simulink model "Non_WindFarm"  (R2024a)
settings: Solver=ode45  StartTime=parSimulacio.ti  StopTime=200  MaxStep=parSimulacio.pas  RelTol=1e-6  AbsTol=1e-6  EnableMultiTasking=on
model workspace (MAT data in the model file):
  tt_vw : Simulink.Parameter (value not decoded)
values from neighbouring files (symbols this model uses):
  L = L'    [Lin_SignalGenerator.m]    (also in Non_ParameterInitialize.m; cal_QR.m = zeros(v, 1); parameters_windFarm2.m)
  nu = size(S, 1)    [Lin_SignalGenerator.m]    (also in Non_ParameterInitialize.m; parameters_windFarm2.m)
  S = zeros(v, v)    [cal_QR.m]
  w0 = [1 -0.00962521549583 0.0254779042049 -0.0160197396127 -0.0156056332727 0.0112137208272 0.0440607583301 -0.0193704893312 -0.0229464276306 -0.00247675309015 0.0285830611299]    [w0.mat]
undefined symbols (not defined in the file or in its folder): parControl, parConvertidor, parGenerador, parGrid, parMecanica, parSimulacio, windspeed
(part 39 of 40)

== system Non_WindFarm/FOM/Wind Farm/Wind Turbine Strings/String6/WT10/WFG/Maquina Sincrona/Park ==
  note: Page 24 eq 3.12
  theta_r : Inport
  Constant4 : Constant  Value=2*pi/3
  Gain7 : Gain  Gain=2/3
  Matrix Concatenate1 : Concatenate  NumInputs=3  Mode=Multidimensional array  ConcatenateDimension=2
  Matrix Concatenate2 : Concatenate  Mode=Multidimensional array  ConcatenateDimension=2
  Mux2 : Mux  Inputs=2
  Mux3 : Mux  Inputs=2
  Mux4 : Mux  Inputs=2
  Mux5 : Mux  Inputs=3
  Mux6 : Mux  Inputs=3
  Sum1 : Sum  Inputs=|++
  Sum2 : Sum  Inputs=|+-
  Trigonometric Function : Trigonometry  Operator=cos
  Trigonometric Function1 : Trigonometry
  Trigonometric Function2 : Trigonometry  Operator=cos
  Trigonometric Function3 : Trigonometry
  Trigonometric Function4 : Trigonometry  Operator=cos
  Trigonometric Function5 : Trigonometry
  Tthetar : Outport
  nTthetar : Outport  Port=2
  wires:
  Constant4/1 -> Sum2/2, Sum1/2
  Trigonometric Function/1 -> Mux2/1, Mux5/1
  Trigonometric Function1/1 -> Mux2/2, Mux6/1
  Trigonometric Function2/1 -> Mux3/1, Mux5/2
  Trigonometric Function3/1 -> Mux3/2, Mux6/2
  Trigonometric Function4/1 -> Mux4/1, Mux5/3
  Trigonometric Function5/1 -> Mux4/2, Mux6/3
  Mux2/1 -> Matrix Concatenate1/1
  Mux3/1 -> Matrix Concatenate1/2
  Mux4/1 -> Matrix Concatenate1/3
  Matrix Concatenate1/1 -> Gain7/1
  Mux5/1 -> Matrix Concatenate2/1
  Mux6/1 -> Matrix Concatenate2/2
  Gain7/1 -> Tthetar/1
  Matrix Concatenate2/1 -> nTthetar/1
  theta_r/1 -> Sum1/1, Sum2/1, Trigonometric Function1/1, Trigonometric Function/1
  Sum2/1 -> Trigonometric Function3/1, Trigonometric Function2/1
  Sum1/1 -> Trigonometric Function5/1, Trigonometric Function4/1

== system Non_WindFarm/FOM/Wind Farm/Wind Turbine Strings/String6/WT10/WFG/Mecanica nolineal i vent/Turbina ==
  note: Page 8
  note: Gamma_t-Wind turbine torque
  note: Wt-turbine speed
  note: Vw-wind speed
  note: Beta-pitch angle
  velocitat_vent : Inport
  omega_aleps : Inport  Port=2
  theta_aleps : Inport  Port=3
  Calcula_Cp : Fcn  Expr=c1*(c2*u[1]-c3*u[2]-c4*u[2]^c5-c6)*exp(-c7*u[1])
  Calcula_parell : Fcn  Expr=u[1]*rho*A*u[2]^3/(2*u[3])
  LAMBDA_inversa : Fcn  Expr=1/(u[1]+c8*u[2])-c9/(1+u[2]^3)
  Mux : Mux  Inputs=2
  Mux1 : Mux  Inputs=2
  Mux2 : Mux  Inputs=2
  Mux3 : Mux  Inputs=3
  calcula_lambda : Fcn  Expr=u[2]*R/u[1]
  parell_turbina : Outport
  Cp : Outport  Port=2
  wires:
  Mux1/1 -> calcula_lambda/1
  omega_aleps/1 -> Mux1/2, Mux3/3
  velocitat_vent/1 -> Mux1/1, Mux3/2
  calcula_lambda/1 -> Mux/1
  theta_aleps/1 -> Mux/2, Mux2/2
  Mux/1 -> LAMBDA_inversa/1
  LAMBDA_inversa/1 -> Mux2/1
  Mux2/1 -> Calcula_Cp/1
  Calcula_Cp/1 -> Mux3/1, Cp/1
  Mux3/1 -> Calcula_parell/1
  Calcula_parell/1 -> parell_turbina/1

== system Non_WindFarm/FOM/Wind Farm/Wind Turbine Strings/String6/WT2/Transformer-complex/homopolar sequence/Park ==
  theta_r : Inport
  Constant4 : Constant  Value=2*pi/3
  Gain7 : Gain  Gain=2/3
  Matrix Concatenate1 : Concatenate  NumInputs=3  Mode=Multidimensional array  ConcatenateDimension=2
  Matrix Concatenate2 : Concatenate  Mode=Multidimensional array  ConcatenateDimension=2
  Mux2 : Mux  Inputs=2
  Mux3 : Mux  Inputs=2
  Mux4 : Mux  Inputs=2
  Mux5 : Mux  Inputs=3
  Mux6 : Mux  Inputs=3
  Sum1 : Sum  Inputs=|++
  Sum2 : Sum  Inputs=|+-
  Trigonometric Function : Trigonometry  Operator=cos
  Trigonometric Function1 : Trigonometry
  Trigonometric Function2 : Trigonometry  Operator=cos
  Trigonometric Function3 : Trigonometry
  Trigonometric Function4 : Trigonometry  Operator=cos
  Trigonometric Function5 : Trigonometry
  Tthetar : Outport
  nTthetar : Outport  Port=2
  wires:
  theta_r/1 -> Sum1/1, Sum2/1, Trigonometric Function/1, Trigonometric Function1/1
  Sum2/1 -> Trigonometric Function2/1, Trigonometric Function3/1
  Sum1/1 -> Trigonometric Function4/1, Trigonometric Function5/1
  Constant4/1 -> Sum2/2, Sum1/2
  Trigonometric Function/1 -> Mux2/1, Mux5/1
  Trigonometric Function1/1 -> Mux2/2, Mux6/1
  Trigonometric Function2/1 -> Mux3/1, Mux5/2
  Trigonometric Function3/1 -> Mux3/2, Mux6/2
  Trigonometric Function4/1 -> Mux4/1, Mux5/3
  Trigonometric Function5/1 -> Mux4/2, Mux6/3
  Mux2/1 -> Matrix Concatenate1/1
  Mux3/1 -> Matrix Concatenate1/2
  Mux4/1 -> Matrix Concatenate1/3
  Matrix Concatenate1/1 -> Gain7/1
  Mux5/1 -> Matrix Concatenate2/1
  Mux6/1 -> Matrix Concatenate2/2
  Gain7/1 -> Tthetar/1
  Matrix Concatenate2/1 -> nTthetar/1

== system Non_WindFarm/FOM/Wind Farm/Wind Turbine Strings/String6/WT2/Transformer-complex/homopolar sequence/homopolar sequence 1 ==
  note: 1/3*v0
  v : Inport
  Add5 : Sum  Inputs=-+
  Constant : Constant  Value=1/3*ones(3)
  Product3 : Product  Multiplication=Matrix(*)  RndMeth=Zero
  v_bar : Outport
  wires:
  Add5/1 -> v_bar/1
  Product3/1 -> Add5/1
  Constant/1 -> Product3/1
  v/1 -> Product3/2, Add5/2

== system Non_WindFarm/FOM/Wind Farm/Wind Turbine Strings/String6/WT2/Transformer-complex/homopolar sequence/homopolar sequence 2 ==
  note: 1/3*v0
  v : Inport
  Add5 : Sum  Inputs=-+
  Constant : Constant  Value=[1/9,1/9,1/9;1/9,1/9,1/9;1/9,1/9,1/9]
  Product3 : Product  Multiplication=Matrix(*)  RndMeth=Zero
  v_bar : Outport
  wires:
  Add5/1 -> v_bar/1
  Product3/1 -> Add5/1
  Constant/1 -> Product3/1
  v/1 -> Product3/2, Add5/2

== system Non_WindFarm/FOM/Wind Farm/Wind Turbine Strings/String6/WT2/WFG/Control Electric Generador/PI ==
  e : Inport
  Demux : Demux  Outputs=2
  Mux2 : Mux  Inputs=2
  Transfer Fcn : TransferFcn  Numerator=[qKp qKi]  Denominator=[1 0]
  Transfer Fcn1 : TransferFcn  Numerator=[dKp dKi]  Denominator=[1 0]
  u : Outport
  wires:
  Transfer Fcn/1 -> Mux2/1
  Transfer Fcn1/1 -> Mux2/2
  Demux/1 -> Transfer Fcn/1
  Demux/2 -> Transfer Fcn1/1
  e/1 -> Demux/1
  Mux2/1 -> u/1

== system Non_WindFarm/FOM/Wind Farm/Wind Turbine Strings/String6/WT2/WFG/Control Electric Generador/Park ==
  theta_r : Inport
  Constant4 : Constant  Value=2*pi/3
  Gain7 : Gain  Gain=2/3
  Matrix Concatenate1 : Concatenate  NumInputs=3  Mode=Multidimensional array  ConcatenateDimension=2
  Matrix Concatenate2 : Concatenate  Mode=Multidimensional array  ConcatenateDimension=2
  Mux2 : Mux  Inputs=2
  Mux3 : Mux  Inputs=2
  Mux4 : Mux  Inputs=2
  Mux5 : Mux  Inputs=3
  Mux6 : Mux  Inputs=3
  Sum1 : Sum  Inputs=|++
  Sum2 : Sum  Inputs=|+-
  Trigonometric Function : Trigonometry  Operator=cos
  Trigonometric Function1 : Trigonometry
  Trigonometric Function2 : Trigonometry  Operator=cos
  Trigonometric Function3 : Trigonometry
  Trigonometric Function4 : Trigonometry  Operator=cos
  Trigonometric Function5 : Trigonometry
  Tthetar : Outport
  nTthetar : Outport  Port=2
  wires:
  theta_r/1 -> Sum1/1, Sum2/1, Trigonometric Function/1, Trigonometric Function1/1
  Sum2/1 -> Trigonometric Function2/1, Trigonometric Function3/1
  Sum1/1 -> Trigonometric Function4/1, Trigonometric Function5/1
  Constant4/1 -> Sum2/2, Sum1/2
  Trigonometric Function/1 -> Mux2/1, Mux5/1
  Trigonometric Function1/1 -> Mux2/2, Mux6/1
  Trigonometric Function2/1 -> Mux3/1, Mux5/2
  Trigonometric Function3/1 -> Mux3/2, Mux6/2
  Trigonometric Function4/1 -> Mux4/1, Mux5/3
  Trigonometric Function5/1 -> Mux4/2, Mux6/3
  Mux2/1 -> Matrix Concatenate1/1
  Mux3/1 -> Matrix Concatenate1/2
  Mux4/1 -> Matrix Concatenate1/3
  Matrix Concatenate1/1 -> Gain7/1
  Mux5/1 -> Matrix Concatenate2/1
  Mux6/1 -> Matrix Concatenate2/2
  Gain7/1 -> Tthetar/1
  Matrix Concatenate2/1 -> nTthetar/1

== system Non_WindFarm/FOM/Wind Farm/Wind Turbine Strings/String6/WT2/WFG/Control Electric Generador/Sat inf ==
  in : Inport
  Abs : Abs  SaturateOnIntegerOverflow=off
  Constant3 : Constant  Value=0.01
  Relational Operator : RelationalOperator  Operator=>  OutDataTypeStr=boolean  InputSameDT=off
  Switch : Switch  Criteria=u2 > Threshold  SaturateOnIntegerOverflow=off  InputSameDT=off
  out : Outport
  wires:
  Abs/1 -> Relational Operator/1
  Constant3/1 -> Relational Operator/2, Switch/3
  Relational Operator/1 -> Switch/2
  in/1 -> Abs/1, Switch/1
  Switch/1 -> out/1

== system Non_WindFarm/FOM/Wind Farm/Wind Turbine Strings/String6/WT2/WFG/Control de Corrent de Xarxa2/PI_d ==
  e : Inport
  Demux : Demux  Outputs=2
  Mux2 : Mux  Inputs=2
  Transfer Fcn : TransferFcn  Numerator=[Kp Ki]  Denominator=[1,0]
  Transfer Fcn1 : TransferFcn  Numerator=[Kp Ki]  Denominator=[1,0]
  u : Outport
  wires:
  Transfer Fcn/1 -> Mux2/1
  Transfer Fcn1/1 -> Mux2/2
  Demux/1 -> Transfer Fcn/1
  Demux/2 -> Transfer Fcn1/1
  e/1 -> Demux/1
  Mux2/1 -> u/1

== system Non_WindFarm/FOM/Wind Farm/Wind Turbine Strings/String6/WT2/WFG/Control de Corrent de Xarxa2/rotacio1 ==
  theta : Inport
  Constant1 : Constant  Value=2*pi/3
  Gain1 : Gain  Gain=-1
  Matrix Concatenate1 : Concatenate  Mode=Multidimensional array  ConcatenateDimension=2
  Matrix Concatenate2 : Concatenate  Mode=Multidimensional array  ConcatenateDimension=2
  Mux1 : Mux  Inputs=3
  Mux2 : Mux  Inputs=2
  Mux3 : Mux  Inputs=2
  Mux5 : Mux  Inputs=3
  Sum4 : Sum  Inputs=|+-
  Sum5 : Sum  Inputs=|++
  Sum6 : Sum  Inputs=|+-
  Sum7 : Sum  Inputs=|++
  Trigonometric Function{,6,8,10} (4 alike) : Trigonometry  Operator=cos
  Trigonometric Function{1,7,9,11} (4 alike) : Trigonometry
  T : Outport
  nT : Outport  Port=2
  wires:
  Trigonometric Function/1 -> Mux2/1, Mux3/2
  Trigonometric Function1/1 -> Gain1/1, Mux2/2
  Mux2/1 -> Matrix Concatenate1/1
  Mux3/1 -> Matrix Concatenate1/2
  Matrix Concatenate1/1 -> T/1
  Matrix Concatenate2/1 -> nT/1
  theta/1 -> Trigonometric Function6/1, Sum4/1, Sum5/1, Trigonometric Function9/1, Sum6/1, Sum7/1, Trigonometric Function/1, Trigonometric Function1/1
  Sum4/1 -> Trigonometric Function10/1
  Constant1/1 -> Sum4/2, Sum5/2, Sum6/2, Sum7/2
  Sum5/1 -> Trigonometric Function8/1
  Sum6/1 -> Trigonometric Function7/1
  Sum7/1 -> Trigonometric Function11/1
  Trigonometric Function6/1 -> Mux5/1
  Trigonometric Function10/1 -> Mux5/2
  Trigonometric Function8/1 -> Mux5/3
  Trigonometric Function9/1 -> Mux1/1
  Trigonometric Function7/1 -> Mux1/2
  Trigonometric Function11/1 -> Mux1/3
  Mux5/1 -> Matrix Concatenate2/1
  Mux1/1 -> Matrix Concatenate2/2
  Gain1/1 -> Mux3/1

== system Non_WindFarm/FOM/Wind Farm/Wind Turbine Strings/String6/WT2/WFG/Maquina Sincrona/Park ==
  note: Page 24 eq 3.12
  theta_r : Inport
  Constant4 : Constant  Value=2*pi/3
  Gain7 : Gain  Gain=2/3
  Matrix Concatenate1 : Concatenate  NumInputs=3  Mode=Multidimensional array  ConcatenateDimension=2
  Matrix Concatenate2 : Concatenate  Mode=Multidimensional array  ConcatenateDimension=2
  Mux2 : Mux  Inputs=2
  Mux3 : Mux  Inputs=2
  Mux4 : Mux  Inputs=2
  Mux5 : Mux  Inputs=3
  Mux6 : Mux  Inputs=3
  Sum1 : Sum  Inputs=|++
  Sum2 : Sum  Inputs=|+-
  Trigonometric Function : Trigonometry  Operator=cos
  Trigonometric Function1 : Trigonometry
  Trigonometric Function2 : Trigonometry  Operator=cos
  Trigonometric Function3 : Trigonometry
  Trigonometric Function4 : Trigonometry  Operator=cos
  Trigonometric Function5 : Trigonometry
  Tthetar : Outport
  nTthetar : Outport  Port=2
  wires:
  Constant4/1 -> Sum2/2, Sum1/2
  Trigonometric Function/1 -> Mux2/1, Mux5/1
  Trigonometric Function1/1 -> Mux2/2, Mux6/1
  Trigonometric Function2/1 -> Mux3/1, Mux5/2
  Trigonometric Function3/1 -> Mux3/2, Mux6/2
  Trigonometric Function4/1 -> Mux4/1, Mux5/3
  Trigonometric Function5/1 -> Mux4/2, Mux6/3
  Mux2/1 -> Matrix Concatenate1/1
  Mux3/1 -> Matrix Concatenate1/2
  Mux4/1 -> Matrix Concatenate1/3
  Matrix Concatenate1/1 -> Gain7/1
  Mux5/1 -> Matrix Concatenate2/1
  Mux6/1 -> Matrix Concatenate2/2
  Gain7/1 -> Tthetar/1
  Matrix Concatenate2/1 -> nTthetar/1
  theta_r/1 -> Sum1/1, Sum2/1, Trigonometric Function1/1, Trigonometric Function/1
  Sum2/1 -> Trigonometric Function3/1, Trigonometric Function2/1
  Sum1/1 -> Trigonometric Function5/1, Trigonometric Function4/1

== system Non_WindFarm/FOM/Wind Farm/Wind Turbine Strings/String6/WT2/WFG/Mecanica nolineal i vent/Turbina ==
  note: Page 8
  note: Gamma_t-Wind turbine torque
  note: Wt-turbine speed
  note: Vw-wind speed
  note: Beta-pitch angle
  velocitat_vent : Inport
  omega_aleps : Inport  Port=2
  theta_aleps : Inport  Port=3
  Calcula_Cp : Fcn  Expr=c1*(c2*u[1]-c3*u[2]-c4*u[2]^c5-c6)*exp(-c7*u[1])
  Calcula_parell : Fcn  Expr=u[1]*rho*A*u[2]^3/(2*u[3])
  LAMBDA_inversa : Fcn  Expr=1/(u[1]+c8*u[2])-c9/(1+u[2]^3)
  Mux : Mux  Inputs=2
  Mux1 : Mux  Inputs=2
  Mux2 : Mux  Inputs=2
  Mux3 : Mux  Inputs=3
  calcula_lambda : Fcn  Expr=u[2]*R/u[1]
  parell_turbina : Outport
  Cp : Outport  Port=2
  wires:
  Mux1/1 -> calcula_lambda/1
  omega_aleps/1 -> Mux1/2, Mux3/3
  velocitat_vent/1 -> Mux1/1, Mux3/2
  calcula_lambda/1 -> Mux/1
  theta_aleps/1 -> Mux/2, Mux2/2
  Mux/1 -> LAMBDA_inversa/1
  LAMBDA_inversa/1 -> Mux2/1
  Mux2/1 -> Calcula_Cp/1
  Calcula_Cp/1 -> Mux3/1, Cp/1
  Mux3/1 -> Calcula_parell/1
  Calcula_parell/1 -> parell_turbina/1

== system Non_WindFarm/FOM/Wind Farm/Wind Turbine Strings/String6/WT3/Transformer-complex/homopolar sequence/Park ==
  theta_r : Inport
  Constant4 : Constant  Value=2*pi/3
  Gain7 : Gain  Gain=2/3
  Matrix Concatenate1 : Concatenate  NumInputs=3  Mode=Multidimensional array  ConcatenateDimension=2
  Matrix Concatenate2 : Concatenate  Mode=Multidimensional array  ConcatenateDimension=2
  Mux2 : Mux  Inputs=2
  Mux3 : Mux  Inputs=2
  Mux4 : Mux  Inputs=2
  Mux5 : Mux  Inputs=3
  Mux6 : Mux  Inputs=3
  Sum1 : Sum  Inputs=|++
  Sum2 : Sum  Inputs=|+-
  Trigonometric Function : Trigonometry  Operator=cos
  Trigonometric Function1 : Trigonometry
  Trigonometric Function2 : Trigonometry  Operator=cos
  Trigonometric Function3 : Trigonometry
  Trigonometric Function4 : Trigonometry  Operator=cos
  Trigonometric Function5 : Trigonometry
  Tthetar : Outport
  nTthetar : Outport  Port=2
  wires:
  Matrix Concatenate2/1 -> nTthetar/1
  Gain7/1 -> Tthetar/1
  Mux6/1 -> Matrix Concatenate2/2
  Mux5/1 -> Matrix Concatenate2/1
  Matrix Concatenate1/1 -> Gain7/1
  Mux4/1 -> Matrix Concatenate1/3
  Mux3/1 -> Matrix Concatenate1/2
  Mux2/1 -> Matrix Concatenate1/1
  Trigonometric Function5/1 -> Mux6/3, Mux4/2
  Trigonometric Function4/1 -> Mux5/3, Mux4/1
  Trigonometric Function3/1 -> Mux6/2, Mux3/2
  Trigonometric Function2/1 -> Mux5/2, Mux3/1
  Trigonometric Function1/1 -> Mux6/1, Mux2/2
  Trigonometric Function/1 -> Mux5/1, Mux2/1
  Constant4/1 -> Sum1/2, Sum2/2
  Sum1/1 -> Trigonometric Function5/1, Trigonometric Function4/1
  Sum2/1 -> Trigonometric Function3/1, Trigonometric Function2/1
  theta_r/1 -> Trigonometric Function1/1, Trigonometric Function/1, Sum2/1, Sum1/1

== system Non_WindFarm/FOM/Wind Farm/Wind Turbine Strings/String6/WT3/Transformer-complex/homopolar sequence/homopolar sequence 1 ==
  note: 1/3*v0
  v : Inport
  Add5 : Sum  Inputs=-+
  Constant : Constant  Value=1/3*ones(3)
  Product3 : Product  Multiplication=Matrix(*)  RndMeth=Zero
  v_bar : Outport
  wires:
  v/1 -> Add5/2, Product3/2
  Constant/1 -> Product3/1
  Product3/1 -> Add5/1
  Add5/1 -> v_bar/1

== system Non_WindFarm/FOM/Wind Farm/Wind Turbine Strings/String6/WT3/Transformer-complex/homopolar sequence/homopolar sequence 2 ==
  note: 1/3*v0
  v : Inport
  Add5 : Sum  Inputs=-+
  Constant : Constant  Value=[1/9,1/9,1/9;1/9,1/9,1/9;1/9,1/9,1/9]
  Product3 : Product  Multiplication=Matrix(*)  RndMeth=Zero
  v_bar : Outport
  wires:
  v/1 -> Add5/2, Product3/2
  Constant/1 -> Product3/1
  Product3/1 -> Add5/1
  Add5/1 -> v_bar/1

== system Non_WindFarm/FOM/Wind Farm/Wind Turbine Strings/String6/WT3/WFG/Control Electric Generador/PI ==
  e : Inport
  Demux : Demux  Outputs=2
  Mux2 : Mux  Inputs=2
  Transfer Fcn : TransferFcn  Numerator=[qKp qKi]  Denominator=[1 0]
  Transfer Fcn1 : TransferFcn  Numerator=[dKp dKi]  Denominator=[1 0]
  u : Outport
  wires:
  Transfer Fcn/1 -> Mux2/1
  Transfer Fcn1/1 -> Mux2/2
  Demux/1 -> Transfer Fcn/1
  Demux/2 -> Transfer Fcn1/1
  e/1 -> Demux/1
  Mux2/1 -> u/1

== system Non_WindFarm/FOM/Wind Farm/Wind Turbine Strings/String6/WT3/WFG/Control Electric Generador/Park ==
  theta_r : Inport
  Constant4 : Constant  Value=2*pi/3
  Gain7 : Gain  Gain=2/3
  Matrix Concatenate1 : Concatenate  NumInputs=3  Mode=Multidimensional array  ConcatenateDimension=2
  Matrix Concatenate2 : Concatenate  Mode=Multidimensional array  ConcatenateDimension=2
  Mux2 : Mux  Inputs=2
  Mux3 : Mux  Inputs=2
  Mux4 : Mux  Inputs=2
  Mux5 : Mux  Inputs=3
  Mux6 : Mux  Inputs=3
  Sum1 : Sum  Inputs=|++
  Sum2 : Sum  Inputs=|+-
  Trigonometric Function : Trigonometry  Operator=cos
  Trigonometric Function1 : Trigonometry
  Trigonometric Function2 : Trigonometry  Operator=cos
  Trigonometric Function3 : Trigonometry
  Trigonometric Function4 : Trigonometry  Operator=cos
  Trigonometric Function5 : Trigonometry
  Tthetar : Outport
  nTthetar : Outport  Port=2
  wires:
  theta_r/1 -> Sum1/1, Sum2/1, Trigonometric Function/1, Trigonometric Function1/1
  Sum2/1 -> Trigonometric Function2/1, Trigonometric Function3/1
  Sum1/1 -> Trigonometric Function4/1, Trigonometric Function5/1
  Constant4/1 -> Sum2/2, Sum1/2
  Trigonometric Function/1 -> Mux2/1, Mux5/1
  Trigonometric Function1/1 -> Mux2/2, Mux6/1
  Trigonometric Function2/1 -> Mux3/1, Mux5/2
  Trigonometric Function3/1 -> Mux3/2, Mux6/2
  Trigonometric Function4/1 -> Mux4/1, Mux5/3
  Trigonometric Function5/1 -> Mux4/2, Mux6/3
  Mux2/1 -> Matrix Concatenate1/1
  Mux3/1 -> Matrix Concatenate1/2
  Mux4/1 -> Matrix Concatenate1/3
  Matrix Concatenate1/1 -> Gain7/1
  Mux5/1 -> Matrix Concatenate2/1
  Mux6/1 -> Matrix Concatenate2/2
  Gain7/1 -> Tthetar/1
  Matrix Concatenate2/1 -> nTthetar/1

== system Non_WindFarm/FOM/Wind Farm/Wind Turbine Strings/String6/WT3/WFG/Control Electric Generador/Sat inf ==
  in : Inport
  Abs : Abs  SaturateOnIntegerOverflow=off
  Constant3 : Constant  Value=0.01
  Relational Operator : RelationalOperator  Operator=>  OutDataTypeStr=boolean  InputSameDT=off
  Switch : Switch  Criteria=u2 > Threshold  SaturateOnIntegerOverflow=off  InputSameDT=off
  out : Outport
  wires:
  Abs/1 -> Relational Operator/1
  Constant3/1 -> Relational Operator/2, Switch/3
  Relational Operator/1 -> Switch/2
  in/1 -> Abs/1, Switch/1
  Switch/1 -> out/1

== system Non_WindFarm/FOM/Wind Farm/Wind Turbine Strings/String6/WT3/WFG/Control de Corrent de Xarxa2/PI_d ==
  e : Inport
  Demux : Demux  Outputs=2
  Mux2 : Mux  Inputs=2
  Transfer Fcn : TransferFcn  Numerator=[Kp Ki]  Denominator=[1,0]
  Transfer Fcn1 : TransferFcn  Numerator=[Kp Ki]  Denominator=[1,0]
  u : Outport
  wires:
  Transfer Fcn/1 -> Mux2/1
  Transfer Fcn1/1 -> Mux2/2
  Demux/1 -> Transfer Fcn/1
  Demux/2 -> Transfer Fcn1/1
  e/1 -> Demux/1
  Mux2/1 -> u/1

== system Non_WindFarm/FOM/Wind Farm/Wind Turbine Strings/String6/WT3/WFG/Control de Corrent de Xarxa2/rotacio1 ==
  theta : Inport
  Constant1 : Constant  Value=2*pi/3
  Gain1 : Gain  Gain=-1
  Matrix Concatenate1 : Concatenate  Mode=Multidimensional array  ConcatenateDimension=2
  Matrix Concatenate2 : Concatenate  Mode=Multidimensional array  ConcatenateDimension=2
  Mux1 : Mux  Inputs=3
  Mux2 : Mux  Inputs=2
  Mux3 : Mux  Inputs=2
  Mux5 : Mux  Inputs=3
  Sum4 : Sum  Inputs=|+-
  Sum5 : Sum  Inputs=|++
  Sum6 : Sum  Inputs=|+-
  Sum7 : Sum  Inputs=|++
  Trigonometric Function{,6,8,10} (4 alike) : Trigonometry  Operator=cos
  Trigonometric Function{1,7,9,11} (4 alike) : Trigonometry
  T : Outport
  nT : Outport  Port=2
  wires:
  Trigonometric Function/1 -> Mux2/1, Mux3/2
  Trigonometric Function1/1 -> Gain1/1, Mux2/2
  Mux2/1 -> Matrix Concatenate1/1
  Mux3/1 -> Matrix Concatenate1/2
  Matrix Concatenate1/1 -> T/1
  Matrix Concatenate2/1 -> nT/1
  theta/1 -> Trigonometric Function6/1, Sum4/1, Sum5/1, Trigonometric Function9/1, Sum6/1, Sum7/1, Trigonometric Function/1, Trigonometric Function1/1
  Sum4/1 -> Trigonometric Function10/1
  Constant1/1 -> Sum4/2, Sum5/2, Sum6/2, Sum7/2
  Sum5/1 -> Trigonometric Function8/1
  Sum6/1 -> Trigonometric Function7/1
  Sum7/1 -> Trigonometric Function11/1
  Trigonometric Function6/1 -> Mux5/1
  Trigonometric Function10/1 -> Mux5/2
  Trigonometric Function8/1 -> Mux5/3
  Trigonometric Function9/1 -> Mux1/1
  Trigonometric Function7/1 -> Mux1/2
  Trigonometric Function11/1 -> Mux1/3
  Mux5/1 -> Matrix Concatenate2/1
  Mux1/1 -> Matrix Concatenate2/2
  Gain1/1 -> Mux3/1

== system Non_WindFarm/FOM/Wind Farm/Wind Turbine Strings/String6/WT3/WFG/Maquina Sincrona/Park ==
  note: Page 24 eq 3.12
  theta_r : Inport
  Constant4 : Constant  Value=2*pi/3
  Gain7 : Gain  Gain=2/3
  Matrix Concatenate1 : Concatenate  NumInputs=3  Mode=Multidimensional array  ConcatenateDimension=2
  Matrix Concatenate2 : Concatenate  Mode=Multidimensional array  ConcatenateDimension=2
  Mux2 : Mux  Inputs=2
  Mux3 : Mux  Inputs=2
  Mux4 : Mux  Inputs=2
  Mux5 : Mux  Inputs=3
  Mux6 : Mux  Inputs=3
  Sum1 : Sum  Inputs=|++
  Sum2 : Sum  Inputs=|+-
  Trigonometric Function : Trigonometry  Operator=cos
  Trigonometric Function1 : Trigonometry
  Trigonometric Function2 : Trigonometry  Operator=cos
  Trigonometric Function3 : Trigonometry
  Trigonometric Function4 : Trigonometry  Operator=cos
  Trigonometric Function5 : Trigonometry
  Tthetar : Outport
  nTthetar : Outport  Port=2
  wires:
  Constant4/1 -> Sum2/2, Sum1/2
  Trigonometric Function/1 -> Mux2/1, Mux5/1
  Trigonometric Function1/1 -> Mux2/2, Mux6/1
  Trigonometric Function2/1 -> Mux3/1, Mux5/2
  Trigonometric Function3/1 -> Mux3/2, Mux6/2
  Trigonometric Function4/1 -> Mux4/1, Mux5/3
  Trigonometric Function5/1 -> Mux4/2, Mux6/3
  Mux2/1 -> Matrix Concatenate1/1
  Mux3/1 -> Matrix Concatenate1/2
  Mux4/1 -> Matrix Concatenate1/3
  Matrix Concatenate1/1 -> Gain7/1
  Mux5/1 -> Matrix Concatenate2/1
  Mux6/1 -> Matrix Concatenate2/2
  Gain7/1 -> Tthetar/1
  Matrix Concatenate2/1 -> nTthetar/1
  theta_r/1 -> Sum1/1, Sum2/1, Trigonometric Function1/1, Trigonometric Function/1
  Sum2/1 -> Trigonometric Function3/1, Trigonometric Function2/1
  Sum1/1 -> Trigonometric Function5/1, Trigonometric Function4/1

== system Non_WindFarm/FOM/Wind Farm/Wind Turbine Strings/String6/WT3/WFG/Mecanica nolineal i vent/Turbina ==
  note: Page 8
  note: Gamma_t-Wind turbine torque
  note: Wt-turbine speed
  note: Vw-wind speed
  note: Beta-pitch angle
  velocitat_vent : Inport
  omega_aleps : Inport  Port=2
  theta_aleps : Inport  Port=3
  Calcula_Cp : Fcn  Expr=c1*(c2*u[1]-c3*u[2]-c4*u[2]^c5-c6)*exp(-c7*u[1])
  Calcula_parell : Fcn  Expr=u[1]*rho*A*u[2]^3/(2*u[3])
  LAMBDA_inversa : Fcn  Expr=1/(u[1]+c8*u[2])-c9/(1+u[2]^3)
  Mux : Mux  Inputs=2
  Mux1 : Mux  Inputs=2
  Mux2 : Mux  Inputs=2
  Mux3 : Mux  Inputs=3
  calcula_lambda : Fcn  Expr=u[2]*R/u[1]
  parell_turbina : Outport
  Cp : Outport  Port=2
  wires:
  Mux1/1 -> calcula_lambda/1
  omega_aleps/1 -> Mux1/2, Mux3/3
  velocitat_vent/1 -> Mux1/1, Mux3/2
  calcula_lambda/1 -> Mux/1
  theta_aleps/1 -> Mux/2, Mux2/2
  Mux/1 -> LAMBDA_inversa/1
  LAMBDA_inversa/1 -> Mux2/1
  Mux2/1 -> Calcula_Cp/1
  Calcula_Cp/1 -> Mux3/1, Cp/1
  Mux3/1 -> Calcula_parell/1
  Calcula_parell/1 -> parell_turbina/1

== system Non_WindFarm/FOM/Wind Farm/Wind Turbine Strings/String6/WT4/Transformer-complex/homopolar sequence/Park ==
  theta_r : Inport
  Constant4 : Constant  Value=2*pi/3
  Gain7 : Gain  Gain=2/3
  Matrix Concatenate1 : Concatenate  NumInputs=3  Mode=Multidimensional array  ConcatenateDimension=2
  Matrix Concatenate2 : Concatenate  Mode=Multidimensional array  ConcatenateDimension=2
  Mux2 : Mux  Inputs=2
  Mux3 : Mux  Inputs=2
  Mux4 : Mux  Inputs=2
  Mux5 : Mux  Inputs=3
  Mux6 : Mux  Inputs=3
  Sum1 : Sum  Inputs=|++
  Sum2 : Sum  Inputs=|+-
  Trigonometric Function : Trigonometry  Operator=cos
  Trigonometric Function1 : Trigonometry
  Trigonometric Function2 : Trigonometry  Operator=cos
  Trigonometric Function3 : Trigonometry
  Trigonometric Function4 : Trigonometry  Operator=cos
  Trigonometric Function5 : Trigonometry
  Tthetar : Outport
  nTthetar : Outport  Port=2
  wires:
  theta_r/1 -> Sum1/1, Sum2/1, Trigonometric Function/1, Trigonometric Function1/1
  Sum2/1 -> Trigonometric Function2/1, Trigonometric Function3/1
  Sum1/1 -> Trigonometric Function4/1, Trigonometric Function5/1
  Constant4/1 -> Sum2/2, Sum1/2
  Trigonometric Function/1 -> Mux2/1, Mux5/1
  Trigonometric Function1/1 -> Mux2/2, Mux6/1
  Trigonometric Function2/1 -> Mux3/1, Mux5/2
  Trigonometric Function3/1 -> Mux3/2, Mux6/2
  Trigonometric Function4/1 -> Mux4/1, Mux5/3
  Trigonometric Function5/1 -> Mux4/2, Mux6/3
  Mux2/1 -> Matrix Concatenate1/1
  Mux3/1 -> Matrix Concatenate1/2
  Mux4/1 -> Matrix Concatenate1/3
  Matrix Concatenate1/1 -> Gain7/1
  Mux5/1 -> Matrix Concatenate2/1
  Mux6/1 -> Matrix Concatenate2/2
  Gain7/1 -> Tthetar/1
  Matrix Concatenate2/1 -> nTthetar/1

== system Non_WindFarm/FOM/Wind Farm/Wind Turbine Strings/String6/WT4/Transformer-complex/homopolar sequence/homopolar sequence 1 ==
  note: 1/3*v0
  v : Inport
  Add5 : Sum  Inputs=-+
  Constant : Constant  Value=1/3*ones(3)
  Product3 : Product  Multiplication=Matrix(*)  RndMeth=Zero
  v_bar : Outport
  wires:
  Add5/1 -> v_bar/1
  Product3/1 -> Add5/1
  Constant/1 -> Product3/1
  v/1 -> Product3/2, Add5/2

== system Non_WindFarm/FOM/Wind Farm/Wind Turbine Strings/String6/WT4/Transformer-complex/homopolar sequence/homopolar sequence 2 ==
  note: 1/3*v0
  v : Inport
  Add5 : Sum  Inputs=-+
  Constant : Constant  Value=[1/9,1/9,1/9;1/9,1/9,1/9;1/9,1/9,1/9]
  Product3 : Product  Multiplication=Matrix(*)  RndMeth=Zero
  v_bar : Outport
  wires:
  Add5/1 -> v_bar/1
  Product3/1 -> Add5/1
  Constant/1 -> Product3/1
  v/1 -> Product3/2, Add5/2

== system Non_WindFarm/FOM/Wind Farm/Wind Turbine Strings/String6/WT4/WFG/Control Electric Generador/PI ==
  e : Inport
  Demux : Demux  Outputs=2
  Mux2 : Mux  Inputs=2
  Transfer Fcn : TransferFcn  Numerator=[qKp qKi]  Denominator=[1 0]
  Transfer Fcn1 : TransferFcn  Numerator=[dKp dKi]  Denominator=[1 0]
  u : Outport
  wires:
  Transfer Fcn/1 -> Mux2/1
  Transfer Fcn1/1 -> Mux2/2
  Demux/1 -> Transfer Fcn/1
  Demux/2 -> Transfer Fcn1/1
  e/1 -> Demux/1
  Mux2/1 -> u/1

== system Non_WindFarm/FOM/Wind Farm/Wind Turbine Strings/String6/WT4/WFG/Control Electric Generador/Park ==
  theta_r : Inport
  Constant4 : Constant  Value=2*pi/3
  Gain7 : Gain  Gain=2/3
  Matrix Concatenate1 : Concatenate  NumInputs=3  Mode=Multidimensional array  ConcatenateDimension=2
  Matrix Concatenate2 : Concatenate  Mode=Multidimensional array  ConcatenateDimension=2
  Mux2 : Mux  Inputs=2
  Mux3 : Mux  Inputs=2
  Mux4 : Mux  Inputs=2
  Mux5 : Mux  Inputs=3
  Mux6 : Mux  Inputs=3
  Sum1 : Sum  Inputs=|++
  Sum2 : Sum  Inputs=|+-
  Trigonometric Function : Trigonometry  Operator=cos
  Trigonometric Function1 : Trigonometry
  Trigonometric Function2 : Trigonometry  Operator=cos
  Trigonometric Function3 : Trigonometry
  Trigonometric Function4 : Trigonometry  Operator=cos
  Trigonometric Function5 : Trigonometry
  Tthetar : Outport
  nTthetar : Outport  Port=2
  wires:
  theta_r/1 -> Sum1/1, Sum2/1, Trigonometric Function/1, Trigonometric Function1/1
  Sum2/1 -> Trigonometric Function2/1, Trigonometric Function3/1
  Sum1/1 -> Trigonometric Function4/1, Trigonometric Function5/1
  Constant4/1 -> Sum2/2, Sum1/2
  Trigonometric Function/1 -> Mux2/1, Mux5/1
  Trigonometric Function1/1 -> Mux2/2, Mux6/1
  Trigonometric Function2/1 -> Mux3/1, Mux5/2
  Trigonometric Function3/1 -> Mux3/2, Mux6/2
  Trigonometric Function4/1 -> Mux4/1, Mux5/3
  Trigonometric Function5/1 -> Mux4/2, Mux6/3
  Mux2/1 -> Matrix Concatenate1/1
  Mux3/1 -> Matrix Concatenate1/2
  Mux4/1 -> Matrix Concatenate1/3
  Matrix Concatenate1/1 -> Gain7/1
  Mux5/1 -> Matrix Concatenate2/1
  Mux6/1 -> Matrix Concatenate2/2
  Gain7/1 -> Tthetar/1
  Matrix Concatenate2/1 -> nTthetar/1

== system Non_WindFarm/FOM/Wind Farm/Wind Turbine Strings/String6/WT4/WFG/Control Electric Generador/Sat inf ==
  in : Inport
  Abs : Abs  SaturateOnIntegerOverflow=off
  Constant3 : Constant  Value=0.01
  Relational Operator : RelationalOperator  Operator=>  OutDataTypeStr=boolean  InputSameDT=off
  Switch : Switch  Criteria=u2 > Threshold  SaturateOnIntegerOverflow=off  InputSameDT=off
  out : Outport
  wires:
  Abs/1 -> Relational Operator/1
  Constant3/1 -> Relational Operator/2, Switch/3
  Relational Operator/1 -> Switch/2
  in/1 -> Abs/1, Switch/1
  Switch/1 -> out/1

== system Non_WindFarm/FOM/Wind Farm/Wind Turbine Strings/String6/WT4/WFG/Control de Corrent de Xarxa2/PI_d ==
  e : Inport
  Demux : Demux  Outputs=2
  Mux2 : Mux  Inputs=2
  Transfer Fcn : TransferFcn  Numerator=[Kp Ki]  Denominator=[1,0]
  Transfer Fcn1 : TransferFcn  Numerator=[Kp Ki]  Denominator=[1,0]
  u : Outport
  wires:
  Transfer Fcn/1 -> Mux2/1
  Transfer Fcn1/1 -> Mux2/2
  Demux/1 -> Transfer Fcn/1
  Demux/2 -> Transfer Fcn1/1
  e/1 -> Demux/1
  Mux2/1 -> u/1

== system Non_WindFarm/FOM/Wind Farm/Wind Turbine Strings/String6/WT4/WFG/Control de Corrent de Xarxa2/rotacio1 ==
  theta : Inport
  Constant1 : Constant  Value=2*pi/3
  Gain1 : Gain  Gain=-1
  Matrix Concatenate1 : Concatenate  Mode=Multidimensional array  ConcatenateDimension=2
  Matrix Concatenate2 : Concatenate  Mode=Multidimensional array  ConcatenateDimension=2
  Mux1 : Mux  Inputs=3
  Mux2 : Mux  Inputs=2
  Mux3 : Mux  Inputs=2
  Mux5 : Mux  Inputs=3
  Sum4 : Sum  Inputs=|+-
  Sum5 : Sum  Inputs=|++
  Sum6 : Sum  Inputs=|+-
  Sum7 : Sum  Inputs=|++
  Trigonometric Function{,6,8,10} (4 alike) : Trigonometry  Operator=cos
  Trigonometric Function{1,7,9,11} (4 alike) : Trigonometry
  T : Outport
  nT : Outport  Port=2
  wires:
  Trigonometric Function/1 -> Mux2/1, Mux3/2
  Trigonometric Function1/1 -> Gain1/1, Mux2/2
  Mux2/1 -> Matrix Concatenate1/1
  Mux3/1 -> Matrix Concatenate1/2
  Matrix Concatenate1/1 -> T/1
  Matrix Concatenate2/1 -> nT/1
  theta/1 -> Trigonometric Function6/1, Sum4/1, Sum5/1, Trigonometric Function9/1, Sum6/1, Sum7/1, Trigonometric Function/1, Trigonometric Function1/1
  Sum4/1 -> Trigonometric Function10/1
  Constant1/1 -> Sum4/2, Sum5/2, Sum6/2, Sum7/2
  Sum5/1 -> Trigonometric Function8/1
  Sum6/1 -> Trigonometric Function7/1
  Sum7/1 -> Trigonometric Function11/1
  Trigonometric Function6/1 -> Mux5/1
  Trigonometric Function10/1 -> Mux5/2
  Trigonometric Function8/1 -> Mux5/3
  Trigonometric Function9/1 -> Mux1/1
  Trigonometric Function7/1 -> Mux1/2
  Trigonometric Function11/1 -> Mux1/3
  Mux5/1 -> Matrix Concatenate2/1
  Mux1/1 -> Matrix Concatenate2/2
  Gain1/1 -> Mux3/1

== system Non_WindFarm/FOM/Wind Farm/Wind Turbine Strings/String6/WT4/WFG/Maquina Sincrona/Park ==
  note: Page 24 eq 3.12
  theta_r : Inport
  Constant4 : Constant  Value=2*pi/3
  Gain7 : Gain  Gain=2/3
  Matrix Concatenate1 : Concatenate  NumInputs=3  Mode=Multidimensional array  ConcatenateDimension=2
  Matrix Concatenate2 : Concatenate  Mode=Multidimensional array  ConcatenateDimension=2
  Mux2 : Mux  Inputs=2
  Mux3 : Mux  Inputs=2
  Mux4 : Mux  Inputs=2
  Mux5 : Mux  Inputs=3
  Mux6 : Mux  Inputs=3
  Sum1 : Sum  Inputs=|++
  Sum2 : Sum  Inputs=|+-
  Trigonometric Function : Trigonometry  Operator=cos
  Trigonometric Function1 : Trigonometry
  Trigonometric Function2 : Trigonometry  Operator=cos
  Trigonometric Function3 : Trigonometry
  Trigonometric Function4 : Trigonometry  Operator=cos
  Trigonometric Function5 : Trigonometry
  Tthetar : Outport
  nTthetar : Outport  Port=2
  wires:
  Constant4/1 -> Sum2/2, Sum1/2
  Trigonometric Function/1 -> Mux2/1, Mux5/1
  Trigonometric Function1/1 -> Mux2/2, Mux6/1
  Trigonometric Function2/1 -> Mux3/1, Mux5/2
  Trigonometric Function3/1 -> Mux3/2, Mux6/2
  Trigonometric Function4/1 -> Mux4/1, Mux5/3
  Trigonometric Function5/1 -> Mux4/2, Mux6/3
  Mux2/1 -> Matrix Concatenate1/1
  Mux3/1 -> Matrix Concatenate1/2
  Mux4/1 -> Matrix Concatenate1/3
  Matrix Concatenate1/1 -> Gain7/1
  Mux5/1 -> Matrix Concatenate2/1
  Mux6/1 -> Matrix Concatenate2/2
  Gain7/1 -> Tthetar/1
  Matrix Concatenate2/1 -> nTthetar/1
  theta_r/1 -> Sum1/1, Sum2/1, Trigonometric Function1/1, Trigonometric Function/1
  Sum2/1 -> Trigonometric Function3/1, Trigonometric Function2/1
  Sum1/1 -> Trigonometric Function5/1, Trigonometric Function4/1

== system Non_WindFarm/FOM/Wind Farm/Wind Turbine Strings/String6/WT4/WFG/Mecanica nolineal i vent/Turbina ==
  note: Page 8
  note: Gamma_t-Wind turbine torque
  note: Wt-turbine speed
  note: Vw-wind speed
  note: Beta-pitch angle
  velocitat_vent : Inport
  omega_aleps : Inport  Port=2
  theta_aleps : Inport  Port=3
  Calcula_Cp : Fcn  Expr=c1*(c2*u[1]-c3*u[2]-c4*u[2]^c5-c6)*exp(-c7*u[1])
  Calcula_parell : Fcn  Expr=u[1]*rho*A*u[2]^3/(2*u[3])
  LAMBDA_inversa : Fcn  Expr=1/(u[1]+c8*u[2])-c9/(1+u[2]^3)
  Mux : Mux  Inputs=2
  Mux1 : Mux  Inputs=2
  Mux2 : Mux  Inputs=2
  Mux3 : Mux  Inputs=3
  calcula_lambda : Fcn  Expr=u[2]*R/u[1]
  parell_turbina : Outport
  Cp : Outport  Port=2
  wires:
  Mux1/1 -> calcula_lambda/1
  omega_aleps/1 -> Mux1/2, Mux3/3
  velocitat_vent/1 -> Mux1/1, Mux3/2
  calcula_lambda/1 -> Mux/1
  theta_aleps/1 -> Mux/2, Mux2/2
  Mux/1 -> LAMBDA_inversa/1
  LAMBDA_inversa/1 -> Mux2/1
  Mux2/1 -> Calcula_Cp/1
  Calcula_Cp/1 -> Mux3/1, Cp/1
  Mux3/1 -> Calcula_parell/1
  Calcula_parell/1 -> parell_turbina/1

== system Non_WindFarm/FOM/Wind Farm/Wind Turbine Strings/String6/WT5/Transformer-complex/homopolar sequence/Park ==
  theta_r : Inport
  Constant4 : Constant  Value=2*pi/3
  Gain7 : Gain  Gain=2/3
  Matrix Concatenate1 : Concatenate  NumInputs=3  Mode=Multidimensional array  ConcatenateDimension=2
  Matrix Concatenate2 : Concatenate  Mode=Multidimensional array  ConcatenateDimension=2
  Mux2 : Mux  Inputs=2
  Mux3 : Mux  Inputs=2
  Mux4 : Mux  Inputs=2
  Mux5 : Mux  Inputs=3
  Mux6 : Mux  Inputs=3
  Sum1 : Sum  Inputs=|++
  Sum2 : Sum  Inputs=|+-
  Trigonometric Function : Trigonometry  Operator=cos
  Trigonometric Function1 : Trigonometry
  Trigonometric Function2 : Trigonometry  Operator=cos
  Trigonometric Function3 : Trigonometry
  Trigonometric Function4 : Trigonometry  Operator=cos
  Trigonometric Function5 : Trigonometry
  Tthetar : Outport
  nTthetar : Outport  Port=2
  wires:
  Matrix Concatenate2/1 -> nTthetar/1
  Gain7/1 -> Tthetar/1
  Mux6/1 -> Matrix Concatenate2/2
  Mux5/1 -> Matrix Concatenate2/1
  Matrix Concatenate1/1 -> Gain7/1
  Mux4/1 -> Matrix Concatenate1/3
  Mux3/1 -> Matrix Concatenate1/2
  Mux2/1 -> Matrix Concatenate1/1
  Trigonometric Function5/1 -> Mux6/3, Mux4/2
  Trigonometric Function4/1 -> Mux5/3, Mux4/1
  Trigonometric Function3/1 -> Mux6/2, Mux3/2
  Trigonometric Function2/1 -> Mux5/2, Mux3/1
  Trigonometric Function1/1 -> Mux6/1, Mux2/2
  Trigonometric Function/1 -> Mux5/1, Mux2/1
  Constant4/1 -> Sum1/2, Sum2/2
  Sum1/1 -> Trigonometric Function5/1, Trigonometric Function4/1
  Sum2/1 -> Trigonometric Function3/1, Trigonometric Function2/1
  theta_r/1 -> Trigonometric Function1/1, Trigonometric Function/1, Sum2/1, Sum1/1

== system Non_WindFarm/FOM/Wind Farm/Wind Turbine Strings/String6/WT5/Transformer-complex/homopolar sequence/homopolar sequence 1 ==
  note: 1/3*v0
  v : Inport
  Add5 : Sum  Inputs=-+
  Constant : Constant  Value=1/3*ones(3)
  Product3 : Product  Multiplication=Matrix(*)  RndMeth=Zero
  v_bar : Outport
  wires:
  v/1 -> Add5/2, Product3/2
  Constant/1 -> Product3/1
  Product3/1 -> Add5/1
  Add5/1 -> v_bar/1

== system Non_WindFarm/FOM/Wind Farm/Wind Turbine Strings/String6/WT5/Transformer-complex/homopolar sequence/homopolar sequence 2 ==
  note: 1/3*v0
  v : Inport
  Add5 : Sum  Inputs=-+
  Constant : Constant  Value=[1/9,1/9,1/9;1/9,1/9,1/9;1/9,1/9,1/9]
  Product3 : Product  Multiplication=Matrix(*)  RndMeth=Zero
  v_bar : Outport
  wires:
  v/1 -> Add5/2, Product3/2
  Constant/1 -> Product3/1
  Product3/1 -> Add5/1
  Add5/1 -> v_bar/1

== system Non_WindFarm/FOM/Wind Farm/Wind Turbine Strings/String6/WT5/WFG/Control Electric Generador/PI ==
  e : Inport
  Demux : Demux  Outputs=2
  Mux2 : Mux  Inputs=2
  Transfer Fcn : TransferFcn  Numerator=[qKp qKi]  Denominator=[1 0]
  Transfer Fcn1 : TransferFcn  Numerator=[dKp dKi]  Denominator=[1 0]
  u : Outport
  wires:
  Transfer Fcn/1 -> Mux2/1
  Transfer Fcn1/1 -> Mux2/2
  Demux/1 -> Transfer Fcn/1
  Demux/2 -> Transfer Fcn1/1
  e/1 -> Demux/1
  Mux2/1 -> u/1

== system Non_WindFarm/FOM/Wind Farm/Wind Turbine Strings/String6/WT5/WFG/Control Electric Generador/Park ==
  theta_r : Inport
  Constant4 : Constant  Value=2*pi/3
  Gain7 : Gain  Gain=2/3
  Matrix Concatenate1 : Concatenate  NumInputs=3  Mode=Multidimensional array  ConcatenateDimension=2
  Matrix Concatenate2 : Concatenate  Mode=Multidimensional array  ConcatenateDimension=2
  Mux2 : Mux  Inputs=2
  Mux3 : Mux  Inputs=2
  Mux4 : Mux  Inputs=2
  Mux5 : Mux  Inputs=3
  Mux6 : Mux  Inputs=3
  Sum1 : Sum  Inputs=|++
  Sum2 : Sum  Inputs=|+-
  Trigonometric Function : Trigonometry  Operator=cos
  Trigonometric Function1 : Trigonometry
  Trigonometric Function2 : Trigonometry  Operator=cos
  Trigonometric Function3 : Trigonometry
  Trigonometric Function4 : Trigonometry  Operator=cos
  Trigonometric Function5 : Trigonometry
  Tthetar : Outport
  nTthetar : Outport  Port=2
  wires:
  theta_r/1 -> Sum1/1, Sum2/1, Trigonometric Function/1, Trigonometric Function1/1
  Sum2/1 -> Trigonometric Function2/1, Trigonometric Function3/1
  Sum1/1 -> Trigonometric Function4/1, Trigonometric Function5/1
  Constant4/1 -> Sum2/2, Sum1/2
  Trigonometric Function/1 -> Mux2/1, Mux5/1
  Trigonometric Function1/1 -> Mux2/2, Mux6/1
  Trigonometric Function2/1 -> Mux3/1, Mux5/2
  Trigonometric Function3/1 -> Mux3/2, Mux6/2
  Trigonometric Function4/1 -> Mux4/1, Mux5/3
  Trigonometric Function5/1 -> Mux4/2, Mux6/3
  Mux2/1 -> Matrix Concatenate1/1
  Mux3/1 -> Matrix Concatenate1/2
  Mux4/1 -> Matrix Concatenate1/3
  Matrix Concatenate1/1 -> Gain7/1
  Mux5/1 -> Matrix Concatenate2/1
  Mux6/1 -> Matrix Concatenate2/2
  Gain7/1 -> Tthetar/1
  Matrix Concatenate2/1 -> nTthetar/1

== system Non_WindFarm/FOM/Wind Farm/Wind Turbine Strings/String6/WT5/WFG/Control Electric Generador/Sat inf ==
  in : Inport
  Abs : Abs  SaturateOnIntegerOverflow=off
  Constant3 : Constant  Value=0.01
  Relational Operator : RelationalOperator  Operator=>  OutDataTypeStr=boolean  InputSameDT=off
  Switch : Switch  Criteria=u2 > Threshold  SaturateOnIntegerOverflow=off  InputSameDT=off
  out : Outport
  wires:
  Abs/1 -> Relational Operator/1
  Constant3/1 -> Relational Operator/2, Switch/3
  Relational Operator/1 -> Switch/2
  in/1 -> Abs/1, Switch/1
  Switch/1 -> out/1

== system Non_WindFarm/FOM/Wind Farm/Wind Turbine Strings/String6/WT5/WFG/Control de Corrent de Xarxa2/PI_d ==
  e : Inport
  Demux : Demux  Outputs=2
  Mux2 : Mux  Inputs=2
  Transfer Fcn : TransferFcn  Numerator=[Kp Ki]  Denominator=[1,0]
  Transfer Fcn1 : TransferFcn  Numerator=[Kp Ki]  Denominator=[1,0]
  u : Outport
  wires:
  Transfer Fcn/1 -> Mux2/1
  Transfer Fcn1/1 -> Mux2/2
  Demux/1 -> Transfer Fcn/1
  Demux/2 -> Transfer Fcn1/1
  e/1 -> Demux/1
  Mux2/1 -> u/1

== system Non_WindFarm/FOM/Wind Farm/Wind Turbine Strings/String6/WT5/WFG/Control de Corrent de Xarxa2/rotacio1 ==
  theta : Inport
  Constant1 : Constant  Value=2*pi/3
  Gain1 : Gain  Gain=-1
  Matrix Concatenate1 : Concatenate  Mode=Multidimensional array  ConcatenateDimension=2
  Matrix Concatenate2 : Concatenate  Mode=Multidimensional array  ConcatenateDimension=2
  Mux1 : Mux  Inputs=3
  Mux2 : Mux  Inputs=2
  Mux3 : Mux  Inputs=2
  Mux5 : Mux  Inputs=3
  Sum4 : Sum  Inputs=|+-
  Sum5 : Sum  Inputs=|++
  Sum6 : Sum  Inputs=|+-
  Sum7 : Sum  Inputs=|++
  Trigonometric Function{,6,8,10} (4 alike) : Trigonometry  Operator=cos
  Trigonometric Function{1,7,9,11} (4 alike) : Trigonometry
  T : Outport
  nT : Outport  Port=2
  wires:
  Trigonometric Function/1 -> Mux2/1, Mux3/2
  Trigonometric Function1/1 -> Gain1/1, Mux2/2
  Mux2/1 -> Matrix Concatenate1/1
  Mux3/1 -> Matrix Concatenate1/2
  Matrix Concatenate1/1 -> T/1
  Matrix Concatenate2/1 -> nT/1
  theta/1 -> Trigonometric Function6/1, Sum4/1, Sum5/1, Trigonometric Function9/1, Sum6/1, Sum7/1, Trigonometric Function/1, Trigonometric Function1/1
  Sum4/1 -> Trigonometric Function10/1
  Constant1/1 -> Sum4/2, Sum5/2, Sum6/2, Sum7/2
  Sum5/1 -> Trigonometric Function8/1
  Sum6/1 -> Trigonometric Function7/1
  Sum7/1 -> Trigonometric Function11/1
  Trigonometric Function6/1 -> Mux5/1
  Trigonometric Function10/1 -> Mux5/2
  Trigonometric Function8/1 -> Mux5/3
  Trigonometric Function9/1 -> Mux1/1
  Trigonometric Function7/1 -> Mux1/2
  Trigonometric Function11/1 -> Mux1/3
  Mux5/1 -> Matrix Concatenate2/1
  Mux1/1 -> Matrix Concatenate2/2
  Gain1/1 -> Mux3/1

== system Non_WindFarm/FOM/Wind Farm/Wind Turbine Strings/String6/WT5/WFG/Maquina Sincrona/Park ==
  note: Page 24 eq 3.12
  theta_r : Inport
  Constant4 : Constant  Value=2*pi/3
  Gain7 : Gain  Gain=2/3
  Matrix Concatenate1 : Concatenate  NumInputs=3  Mode=Multidimensional array  ConcatenateDimension=2
  Matrix Concatenate2 : Concatenate  Mode=Multidimensional array  ConcatenateDimension=2
  Mux2 : Mux  Inputs=2
  Mux3 : Mux  Inputs=2
  Mux4 : Mux  Inputs=2
  Mux5 : Mux  Inputs=3
  Mux6 : Mux  Inputs=3
  Sum1 : Sum  Inputs=|++
  Sum2 : Sum  Inputs=|+-
  Trigonometric Function : Trigonometry  Operator=cos
  Trigonometric Function1 : Trigonometry
  Trigonometric Function2 : Trigonometry  Operator=cos
  Trigonometric Function3 : Trigonometry
  Trigonometric Function4 : Trigonometry  Operator=cos
  Trigonometric Function5 : Trigonometry
  Tthetar : Outport
  nTthetar : Outport  Port=2
  wires:
  Constant4/1 -> Sum2/2, Sum1/2
  Trigonometric Function/1 -> Mux2/1, Mux5/1
  Trigonometric Function1/1 -> Mux2/2, Mux6/1
  Trigonometric Function2/1 -> Mux3/1, Mux5/2
  Trigonometric Function3/1 -> Mux3/2, Mux6/2
  Trigonometric Function4/1 -> Mux4/1, Mux5/3
  Trigonometric Function5/1 -> Mux4/2, Mux6/3
  Mux2/1 -> Matrix Concatenate1/1
  Mux3/1 -> Matrix Concatenate1/2
  Mux4/1 -> Matrix Concatenate1/3
  Matrix Concatenate1/1 -> Gain7/1
  Mux5/1 -> Matrix Concatenate2/1
  Mux6/1 -> Matrix Concatenate2/2
  Gain7/1 -> Tthetar/1
  Matrix Concatenate2/1 -> nTthetar/1
  theta_r/1 -> Sum1/1, Sum2/1, Trigonometric Function1/1, Trigonometric Function/1
  Sum2/1 -> Trigonometric Function3/1, Trigonometric Function2/1
  Sum1/1 -> Trigonometric Function5/1, Trigonometric Function4/1

== system Non_WindFarm/FOM/Wind Farm/Wind Turbine Strings/String6/WT5/WFG/Mecanica nolineal i vent/Turbina ==
  note: Page 8
  note: Gamma_t-Wind turbine torque
  note: Wt-turbine speed
  note: Vw-wind speed
  note: Beta-pitch angle
  velocitat_vent : Inport
  omega_aleps : Inport  Port=2
  theta_aleps : Inport  Port=3
  Calcula_Cp : Fcn  Expr=c1*(c2*u[1]-c3*u[2]-c4*u[2]^c5-c6)*exp(-c7*u[1])
  Calcula_parell : Fcn  Expr=u[1]*rho*A*u[2]^3/(2*u[3])
  LAMBDA_inversa : Fcn  Expr=1/(u[1]+c8*u[2])-c9/(1+u[2]^3)
  Mux : Mux  Inputs=2
  Mux1 : Mux  Inputs=2
  Mux2 : Mux  Inputs=2
  Mux3 : Mux  Inputs=3
  calcula_lambda : Fcn  Expr=u[2]*R/u[1]
  parell_turbina : Outport
  Cp : Outport  Port=2
  wires:
  Mux1/1 -> calcula_lambda/1
  omega_aleps/1 -> Mux1/2, Mux3/3
  velocitat_vent/1 -> Mux1/1, Mux3/2
  calcula_lambda/1 -> Mux/1
  theta_aleps/1 -> Mux/2, Mux2/2
  Mux/1 -> LAMBDA_inversa/1
  LAMBDA_inversa/1 -> Mux2/1
  Mux2/1 -> Calcula_Cp/1
  Calcula_Cp/1 -> Mux3/1, Cp/1
  Mux3/1 -> Calcula_parell/1
  Calcula_parell/1 -> parell_turbina/1

== system Non_WindFarm/FOM/Wind Farm/Wind Turbine Strings/String6/WT6/Transformer-complex/homopolar sequence/Park ==
  theta_r : Inport
  Constant4 : Constant  Value=2*pi/3
  Gain7 : Gain  Gain=2/3
  Matrix Concatenate1 : Concatenate  NumInputs=3  Mode=Multidimensional array  ConcatenateDimension=2
  Matrix Concatenate2 : Concatenate  Mode=Multidimensional array  ConcatenateDimension=2
  Mux2 : Mux  Inputs=2
  Mux3 : Mux  Inputs=2
  Mux4 : Mux  Inputs=2
  Mux5 : Mux  Inputs=3
  Mux6 : Mux  Inputs=3
  Sum1 : Sum  Inputs=|++
  Sum2 : Sum  Inputs=|+-
  Trigonometric Function : Trigonometry  Operator=cos
  Trigonometric Function1 : Trigonometry
  Trigonometric Function2 : Trigonometry  Operator=cos
  Trigonometric Function3 : Trigonometry
  Trigonometric Function4 : Trigonometry  Operator=cos
  Trigonometric Function5 : Trigonometry
  Tthetar : Outport
  nTthetar : Outport  Port=2
  wires:
  theta_r/1 -> Sum1/1, Sum2/1, Trigonometric Function/1, Trigonometric Function1/1
  Sum2/1 -> Trigonometric Function2/1, Trigonometric Function3/1
  Sum1/1 -> Trigonometric Function4/1, Trigonometric Function5/1
  Constant4/1 -> Sum2/2, Sum1/2
  Trigonometric Function/1 -> Mux2/1, Mux5/1
  Trigonometric Function1/1 -> Mux2/2, Mux6/1
  Trigonometric Function2/1 -> Mux3/1, Mux5/2
  Trigonometric Function3/1 -> Mux3/2, Mux6/2
  Trigonometric Function4/1 -> Mux4/1, Mux5/3
  Trigonometric Function5/1 -> Mux4/2, Mux6/3
  Mux2/1 -> Matrix Concatenate1/1
  Mux3/1 -> Matrix Concatenate1/2
  Mux4/1 -> Matrix Concatenate1/3
  Matrix Concatenate1/1 -> Gain7/1
  Mux5/1 -> Matrix Concatenate2/1
  Mux6/1 -> Matrix Concatenate2/2
  Gain7/1 -> Tthetar/1
  Matrix Concatenate2/1 -> nTthetar/1

== system Non_WindFarm/FOM/Wind Farm/Wind Turbine Strings/String6/WT6/Transformer-complex/homopolar sequence/homopolar sequence 1 ==
  note: 1/3*v0
  v : Inport
  Add5 : Sum  Inputs=-+
  Constant : Constant  Value=1/3*ones(3)
  Product3 : Product  Multiplication=Matrix(*)  RndMeth=Zero
  v_bar : Outport
  wires:
  Add5/1 -> v_bar/1
  Product3/1 -> Add5/1
  Constant/1 -> Product3/1
  v/1 -> Product3/2, Add5/2

== system Non_WindFarm/FOM/Wind Farm/Wind Turbine Strings/String6/WT6/Transformer-complex/homopolar sequence/homopolar sequence 2 ==
  note: 1/3*v0
  v : Inport
  Add5 : Sum  Inputs=-+
  Constant : Constant  Value=[1/9,1/9,1/9;1/9,1/9,1/9;1/9,1/9,1/9]
  Product3 : Product  Multiplication=Matrix(*)  RndMeth=Zero
  v_bar : Outport
  wires:
  Add5/1 -> v_bar/1
  Product3/1 -> Add5/1
  Constant/1 -> Product3/1
  v/1 -> Product3/2, Add5/2

== system Non_WindFarm/FOM/Wind Farm/Wind Turbine Strings/String6/WT6/WFG/Control Electric Generador/PI ==
  e : Inport
  Demux : Demux  Outputs=2
  Mux2 : Mux  Inputs=2
  Transfer Fcn : TransferFcn  Numerator=[qKp qKi]  Denominator=[1 0]
  Transfer Fcn1 : TransferFcn  Numerator=[dKp dKi]  Denominator=[1 0]
  u : Outport
  wires:
  Transfer Fcn/1 -> Mux2/1
  Transfer Fcn1/1 -> Mux2/2
  Demux/1 -> Transfer Fcn/1
  Demux/2 -> Transfer Fcn1/1
  e/1 -> Demux/1
  Mux2/1 -> u/1

== system Non_WindFarm/FOM/Wind Farm/Wind Turbine Strings/String6/WT6/WFG/Control Electric Generador/Park ==
  theta_r : Inport
  Constant4 : Constant  Value=2*pi/3
  Gain7 : Gain  Gain=2/3
  Matrix Concatenate1 : Concatenate  NumInputs=3  Mode=Multidimensional array  ConcatenateDimension=2
  Matrix Concatenate2 : Concatenate  Mode=Multidimensional array  ConcatenateDimension=2
  Mux2 : Mux  Inputs=2
  Mux3 : Mux  Inputs=2
  Mux4 : Mux  Inputs=2
  Mux5 : Mux  Inputs=3
  Mux6 : Mux  Inputs=3
  Sum1 : Sum  Inputs=|++
  Sum2 : Sum  Inputs=|+-
  Trigonometric Function : Trigonometry  Operator=cos
  Trigonometric Function1 : Trigonometry
  Trigonometric Function2 : Trigonometry  Operator=cos
  Trigonometric Function3 : Trigonometry
  Trigonometric Function4 : Trigonometry  Operator=cos
  Trigonometric Function5 : Trigonometry
  Tthetar : Outport
  nTthetar : Outport  Port=2
  wires:
  theta_r/1 -> Sum1/1, Sum2/1, Trigonometric Function/1, Trigonometric Function1/1
  Sum2/1 -> Trigonometric Function2/1, Trigonometric Function3/1
  Sum1/1 -> Trigonometric Function4/1, Trigonometric Function5/1
  Constant4/1 -> Sum2/2, Sum1/2
  Trigonometric Function/1 -> Mux2/1, Mux5/1
  Trigonometric Function1/1 -> Mux2/2, Mux6/1
  Trigonometric Function2/1 -> Mux3/1, Mux5/2
  Trigonometric Function3/1 -> Mux3/2, Mux6/2
  Trigonometric Function4/1 -> Mux4/1, Mux5/3
  Trigonometric Function5/1 -> Mux4/2, Mux6/3
  Mux2/1 -> Matrix Concatenate1/1
  Mux3/1 -> Matrix Concatenate1/2
  Mux4/1 -> Matrix Concatenate1/3
  Matrix Concatenate1/1 -> Gain7/1
  Mux5/1 -> Matrix Concatenate2/1
  Mux6/1 -> Matrix Concatenate2/2
  Gain7/1 -> Tthetar/1
  Matrix Concatenate2/1 -> nTthetar/1

== system Non_WindFarm/FOM/Wind Farm/Wind Turbine Strings/String6/WT6/WFG/Control Electric Generador/Sat inf ==
  in : Inport
  Abs : Abs  SaturateOnIntegerOverflow=off
  Constant3 : Constant  Value=0.01
  Relational Operator : RelationalOperator  Operator=>  OutDataTypeStr=boolean  InputSameDT=off
  Switch : Switch  Criteria=u2 > Threshold  SaturateOnIntegerOverflow=off  InputSameDT=off
  out : Outport
  wires:
  Abs/1 -> Relational Operator/1
  Constant3/1 -> Relational Operator/2, Switch/3
  Relational Operator/1 -> Switch/2
  in/1 -> Abs/1, Switch/1
  Switch/1 -> out/1

== system Non_WindFarm/FOM/Wind Farm/Wind Turbine Strings/String6/WT6/WFG/Control de Corrent de Xarxa2/PI_d ==
  e : Inport
  Demux : Demux  Outputs=2
  Mux2 : Mux  Inputs=2
  Transfer Fcn : TransferFcn  Numerator=[Kp Ki]  Denominator=[1,0]
  Transfer Fcn1 : TransferFcn  Numerator=[Kp Ki]  Denominator=[1,0]
  u : Outport
  wires:
  Transfer Fcn/1 -> Mux2/1
  Transfer Fcn1/1 -> Mux2/2
  Demux/1 -> Transfer Fcn/1
  Demux/2 -> Transfer Fcn1/1
  e/1 -> Demux/1
  Mux2/1 -> u/1
